simulink model "project2_sim_no_roomba"  (R2017a)
settings: Solver=VariableStepAuto  StartTime=0.0  StopTime=Inf  RelTol=1e-3
libraries: realtime_pacer_lib x1
settings Model: Creator=bai  LastModifiedBy=tuf53749

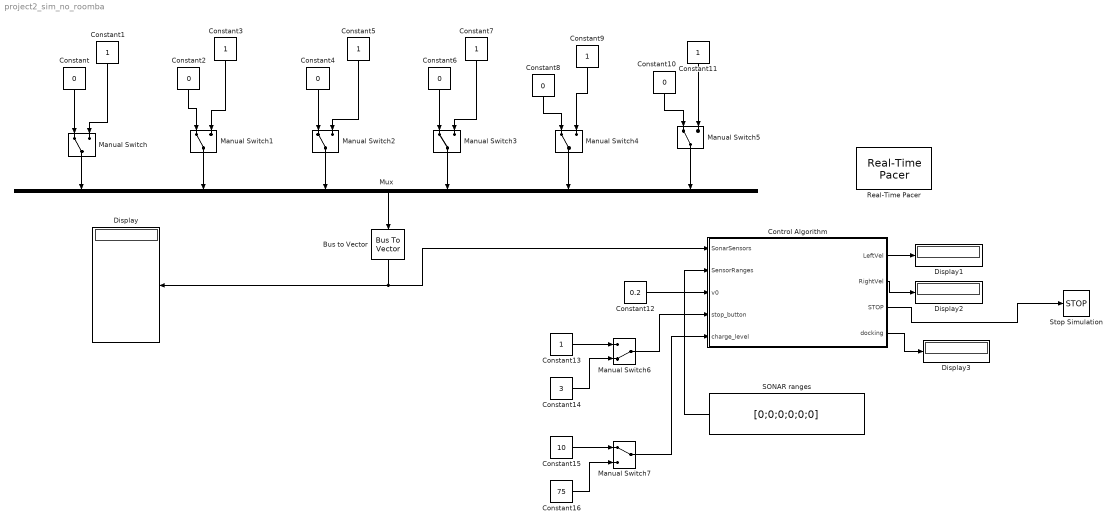
== system project2_sim_no_roomba ==
  Bus to Vector : BusToVector
  Constant{,2,4,6,8,10} (6 alike) : Constant  Value=0
  Constant{1,3,5,7,9,11,13} (7 alike) : Constant
  Constant12 : Constant  Value=0.2
  Constant14 : Constant  Value=3
  Constant15 : Constant  Value=10
  Constant16 : Constant  Value=75
  Control Algorithm : Stateflow chart  TreatAsAtomicUnit=on  mask{v0=1}
      mask prompts: v0 "Wheel Angular Velocity"
  Display{,1..3} (4 alike) : Display
  Manual Switch{,1..5,7} (7 alike) : ManualSwitch
  Manual Switch6 : ManualSwitch  CurrentSetting=0
  Mux : Mux  Inputs=6
  Real-Time Pacer : realtime_pacer_lib/Real-Time Pacer  simTimePerRealTime=1
  SONAR ranges : Constant  Value=[0;0;0;0;0;0]
  Stop Simulation : Stop
  wires:
  Manual Switch1/1 -> Mux/2
  Constant10/1 -> Manual Switch5/1
  Constant2/1 -> Manual Switch1/1
  Constant3/1 -> Manual Switch1/2
  Constant9/1 -> Manual Switch4/2
  Constant7/1 -> Manual Switch3/2
  Manual Switch/1 -> Mux/1
  Constant5/1 -> Manual Switch2/2
  Constant11/1 -> Manual Switch5/2
  SONAR ranges/1 -> Control Algorithm/2(SensorRanges)
  Manual Switch2/1 -> Mux/3
  Constant/1 -> Manual Switch/1
  Manual Switch4/1 -> Mux/5
  Manual Switch3/1 -> Mux/4
  Constant8/1 -> Manual Switch4/1
  Mux/1 -> Bus to Vector/1
  Manual Switch5/1 -> Mux/6
  Bus to Vector/1 -> Display/1, Control Algorithm/1(SonarSensors)
  Constant4/1 -> Manual Switch2/1
  Constant6/1 -> Manual Switch3/1
  Constant1/1 -> Manual Switch/2
  Constant12/1 -> Control Algorithm/3(v0)
  Manual Switch6/1 -> Control Algorithm/4(stop_button)
  Constant13/1 -> Manual Switch6/1
  Constant14/1 -> Manual Switch6/2
  Control Algorithm/3(STOP) -> Stop Simulation/1
  Control Algorithm/1(LeftVel) -> Display1/1
  Control Algorithm/2(RightVel) -> Display2/1
  Constant15/1 -> Manual Switch7/1
  Constant16/1 -> Manual Switch7/2
  Manual Switch7/1 -> Control Algorithm/5(charge_level)
  Control Algorithm/4(docking) -> Display3/1

== stateflow chart project2_sim_no_roomba/Control Algorithm ==
  state BatteryLevelLogic [parallel]
    settings: executionOrder=3
    state CheckBat
      en:
      docking = 0;
    state LowBat
      en:
      docking = 1;
      %SeekDockRoomba_Get();
    (default) -> CheckBat
    CheckBat -> LowBat : [charge_level <= 10]
  state EmergencyStopLogic [parallel]
    settings: executionOrder=1
    state StopButtonOFF
      en:
      %do nothing
      %
      STOP = 0;
    state StopButtonON
      en:
      LeftVel = 0;
      RightVel = 0;
      %this output must be
      %wired to Simulink
      %stop sink block
      %
      STOP = 1;
    (default) -> StopButtonOFF : {STOP=0;}
    StopButtonOFF -> StopButtonOFF [order 2] : after(0.1,sec)
    StopButtonOFF -> StopButtonON [order 1] : [stop_button == 3]
  state ObstacleAvoidLogic [parallel]
    en,du:
    frontSensors = SonarSensors(3:4);
    %frontSensors = SonarSensors(3:4) > SensorRanges(3:4);
    %leftMostSensors = [SonarSensors(1)] > SensorRanges(1);
    %leftMiddleSensors = [SonarSensors(1:2)] > SensorRanges(1:2);
    %rightMiddleSensors = [SonarSensors(5:6)] > SensorRanges(5:6);
    %rightMostSensors = [SonarSensors(6) ]> SensorRanges(6);
    leftMT=[SonarSensors(1)]; %>SensorRanges(1);
    leftMD=[SonarSensors(2)]; %>SensorRanges(2);
    leftFT=[SonarSensors(3)]; %>SensorRanges(3);
    rightFT=[SonarSensors(4)]; %>SensorRanges(4);
    rightMD=[SonarSensors(5)]; %>SensorRanges(5);
    rightMT=[SonarSensors(6)]; %>SensorRanges(6);
    settings: executionOrder=2
    state InitialCount
      en:
      count=0;
    state ReverseABit
      en,du:
      RightVel = -v0;
      LeftVel = -v0;
    state GoStraight
      en,du:
      RightVel = v0;
      LeftVel = v0;
    state TurnRightWide
      du:
      RightVel = v0/2;
      LeftVel = v0;
    state TurnRightTight
      du :
      RightVel = v0/5;
      LeftVel = v0;
    state TurnLeftInPlace
      du :
      RightVel = v0;
      LeftVel = -v0;
    state TurnRightInPlace
      du :
      RightVel = -v0;
      LeftVel = v0;
    state TurnLeftWide
      du :
      RightVel = v0;
      LeftVel = v0/2;
    state TurnLeftTight
      du :
      RightVel = v0;
      LeftVel = v0/5;
    state ReverseABit1
      en,du:
      RightVel = -v0;
      LeftVel = -v0;
    state ReverseALot
      en,du:
      RightVel = -v0;
      LeftVel = -v0;
    state DetermineRightLeft
    state DeterminerightWide
    state DetermineLeftTight
    state Nothing
    state DetermineCount
    state DeterminerightTight
    state DetermineFront
    state DetermineLeftWide
    state Count
      entry:count=count+1;
    state Stop
      en,du:
      RightVel = 0;
      LeftVel = 0;
    (default) -> InitialCount
    InitialCount -> ReverseABit
    ReverseABit -> GoStraight : after(3,sec)
    GoStraight -> DeterminerightWide
    TurnRightWide -> GoStraight : [leftMT<1]
    TurnRightTight -> GoStraight : [leftMT<1&&leftMD<1]
    TurnLeftInPlace -> GoStraight : [rightFT<1&&leftFT<1]
    TurnRightInPlace -> GoStraight : [rightFT<1&&leftFT<1]
    TurnLeftWide -> GoStraight : [rightMT<1]
    TurnLeftTight -> GoStraight : [rightMD<1&&rightMT<1]
    Nothing -> GoStraight [order 1] : [leftMT<1&&...
        | leftMD<1&&...
        | leftFT<1&&...
        | rightFT<1&&...
        | rightMD<1&&...
        | rightMT<1]
    ReverseABit1 -> GoStraight : after(2,sec)
    ReverseALot -> GoStraight : after(6,sec)
    DeterminerightTight -> TurnRightTight [order 1] : [leftMT>0&&...
        | leftMD>0&&...
        | leftFT<1&&...
        | rightFT<1&&...
        | rightMD<1&&...
        | rightMT<1]
    DetermineRightLeft -> TurnLeftInPlace [order 2] : %default
    DetermineRightLeft -> TurnRightInPlace [order 1] : [rightFT>rightMD]
    DetermineLeftWide -> TurnLeftWide [order 1] : [leftMT<1&&...
        | leftMD<1&&...
        | leftFT<1&&...
        | rightFT<1&&...
        | rightMD<1&&...
        | rightMT>0]
    DetermineLeftTight -> TurnLeftTight [order 1] : [leftMT<1&&...
        | leftMD<1&&...
        | leftFT<1&&...
        | rightFT<1&&...
        | rightMD>0&&...
        | rightMT>0]
    DeterminerightWide -> TurnRightWide [order 1] : [leftMT>0&&...
        | leftMD<1&&...
        | leftFT<1&&...
        | rightFT<1&&...
        | rightMD<1&&...
        | rightMT<1]
    DetermineCount -> ReverseABit1 [order 1] : [count<5]
    DetermineCount -> ReverseALot [order 3] : [count<10 && count>5]
    DetermineFront -> DetermineRightLeft [order 1] : [leftMT<1&&...
        | leftMD<1&&leftFT>0&&...
        | rightFT>0&&rightMD<1&&...
        | rightMT<1]
    DeterminerightWide -> DeterminerightTight [order 2] : %default
    DetermineLeftTight -> Nothing [order 2] : %default
    DetermineLeftWide -> DetermineLeftTight [order 2] : %default
    Nothing -> Count [order 2] : %default
    Count -> DetermineCount : %default
    DetermineCount -> Stop [order 2] : [count>10]
    DeterminerightTight -> DetermineFront [order 2] : %default
    DetermineFront -> DetermineLeftWide [order 2] : %default
  data: LeftVel output; RightVel output; SonarSensors input; frontSensors local; SensorRanges input; leftMostSensors local; leftMiddleSensors local; rightMostSensors local; rightMiddleSensors local; rightMT local; leftFT local; rightMD local; rightFT local; leftMD local; leftMT local; count local; v0 input [0..0.5]; stop_button input; STOP output [0..1]; charge_level input; docking output
  function SeekDockRoomba_Get:
    | function SeekDockRoomba_Get
    | persistent obj
    | coder.extrinsic('SeekDockRoomba');
    | coder.extrinsic('evalin');
    | coder.extrinsic('get');
    | if isempty(obj)
    |     obj = evalin('base','objWs');
    | end
    | SeekDockRoomba(obj);
